simulink model "formation"  (Simulink 6.6)
settings: Solver=ode45  StartTime=0.0  StopTime=20  RelTol=1e-3
values from neighbouring files (symbols this model uses):
  A = kron(eye(N),Ai)    [init.m]
  Ai = [0 1 0 0 ... (first row only)    [init.m]
  B = kron(L,Bi*Fi)    [init.m]
  Bi = [0;1;0;1]    [init.m]
  C = eye(size(A))    [init.m]
  Ci = eye(4)    [init.m]
  D = zeros(size(B))    [init.m]
  Di = [0 0 0 0]'    [init.m]
  h = zeros(length(A),1)    [init.m]
  x0 = ones(length(A),1)    [init.m]
  xi0 = [1 0 1 0 ]'    [init.m]
settings Model: Creator=wizest  LastModifiedBy=wizest

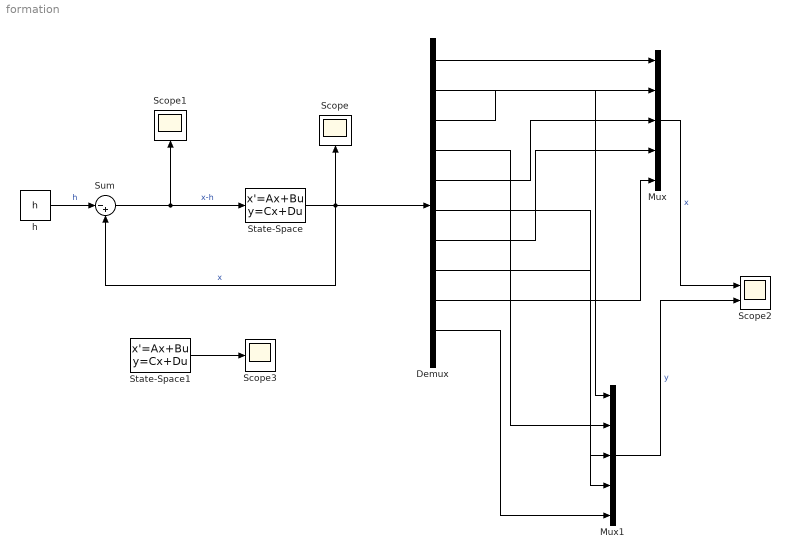
== system formation ==
  Demux : Demux  Outputs=20
  Mux : Mux  Inputs=5
  Mux1 : Mux  Inputs=5
  Scope : Scope
      settings: Orientation=up  TimeRange=20  YMin=0  YMax=25
  Scope1 : Scope
      settings: Orientation=up
  Scope2 : Scope  NumInputPorts=2
      settings: TimeRange=20  YMin=0~0  YMax=25~25  SaveName=ScopeData2
  Scope3 : Scope
      settings: TimeRange=20  YMin=-1  YMax=1  SaveName=ScopeData3
  State-Space : StateSpace  A=A  B=B  C=C  D=D  X0=x0
  State-Space1 : StateSpace  A=Ai  B=Bi  C=Ci  D=Di  X0=xi0
  Sum : Sum  Inputs=|-+
  h : Constant  Value=h
  wires:
  Sum/1 -> State-Space/1, Scope1/1  "x-h"
  h/1 -> Sum/1  "h"
  State-Space/1 -> Sum/2, Demux/1, Scope/1  "x"
  Demux/1 -> Mux/1
  Demux/5 -> Mux/2
  Demux/9 -> Mux/3
  Demux/13 -> Mux/4
  Demux/17 -> Mux/5
  Demux/3 -> Mux1/1
  Demux/7 -> Mux1/2
  Demux/11 -> Mux1/3
  Demux/15 -> Mux1/4
  Demux/19 -> Mux1/5
  Mux/1 -> Scope2/1  "x"
  Mux1/1 -> Scope2/2  "y"
  State-Space1/1 -> Scope3/1
